simulink model "Ej11"  (R2025b)
settings: Solver=VariableStepAuto  StartTime=0.0  StopTime=inf  RelTol=1e-3
libraries: commdigbbndam3 x4, commrandsrc3 x1
settings Model: Creator=Henry  LastModifiedBy=Henry

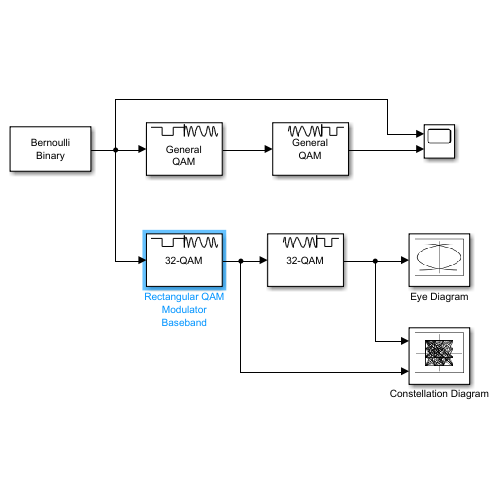
[thumbnail: Simulink's stored preview of the top-level diagram]
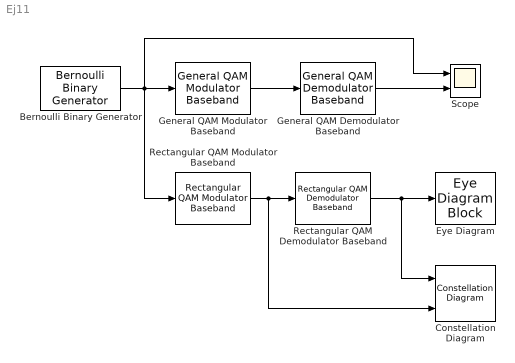
== system Ej11 ==
  Bernoulli Binary Generator : commrandsrc3/Bernoulli Binary Generator  ProbabilityOfZero=0.5  SeedSource=Auto  Seed=0  SampleTime=1  SamplesPerFrame=2  OutputDataType=double  SimulateUsing=Interpreted execution
  Constellation Diagram : ConstellationDiagram  NumInputPorts=2  WindowPosition=[36.000000,127.000000,600.000000,600.000000,]  ScopeFrameLocation=window  SymbolsToDisplay=8  ReferenceConstellation="{[-1.0801+1.0801i         -1.0801+0.77152i         -1.0801+0.46291i          -1.0801+0.1543i          -1.0801-0.1543i         -1.0801-0.46291i         -1.0801-0.77152i          -1.0801-1.0801i         -0.77152+1.0801i        -0.77152+0.77152i        -0.77152+0.46291i         -0.77152+0.1543i         -0.77152-0.1543i        -0.77152-0.46291i        -0.77152-0.77152i         -0.77152-1.0801i         -0.46291+1.0801i        -0.46291+0.77152i        -0.46291+0.46291i         -0.46291+0.1543i         -0.46291-0.1543i        -0.46291-0.46291i        -0.46291-0.77152i         -0.46291-1.0801i          -0.1543+1.0801i         -0.1543+0.77152i         -0.1543+0.46291i          -0.1543+0.1543i          -0.1543-0.1543i         -0.1543-0.46291i         -0.1543-0.77152i          -0.1543-1.0801i           0.1543+1.0801i          0.1543+0.77152i          0.1543+0.46291i           0.1543+0.1543i           0.1543-0.1543i          0.1543-0.46291i          0.1543-0.77152i           0.1543-1.0801i          0.46291+1.0801i         0.46291+0.77152i         0.46291+0.46291i          0.46291+0.1543i          0.46291-0.1543i         0.46291-0.46291i         0.46291-0.77152i          0.46291-1.0801i          0.77152+1.0801i         0.77152+0.77152i         0.77152+0.46291i          0.77152+0.1543i          0.77152-0.1543i         0.77152-0.46291i         0.77152-0.77152i          0.77152-1.0801i           1.0801+1.0801i          1.0801+0.77152i          1.0801+0.46291i           1.0801+0.1543i           1.0801-0.1543i          1.0801-0.46291i          1.0801-0.77152i           1.0801-1.0801i][-1.0801+1.0801i         -1.0801+0.77152i         -1.0801+0.46291i          -1.0801+0.1543i          -1.0801-0.1543i         -1.0801-0.46291i         -1.0801-0.77152i          -1.0801-1.0801i         -0.77152+1.0801i        -0.77152+0.77152i        -0.77152+0.46291i         -0.77152+0.1543i         -0.77152-0.1543i        -0.77152-0.46291i        -0.77152-0.77152i         -0.77152-1.0801i         -0.46291+1.0801i        -0.46291+0.77152i        -0.46291+0.46291i         -0.46291+0.1543i         -0.46291-0.1543i        -0.46291-0.46291i        -0.46291-0.77152i         -0.46291-1.0801i          -0.1543+1.0801i         -0.1543+0.77152i         -0.1543+0.46291i          -0.1543+0.1543i          -0.1543-0.1543i         -0.1543-0.46291i         -0.1543-0.77152i          -0.1543-1.0801i           0.1543+1.0801i          0.1543+0.77152i          0.1543+0.46291i           0.1543+0.1543i           0.1543-0.1543i          0.1543-0.46291i          0.1543-0.77152i           0.1543-1.0801i          0.46291+1.0801i         0.46291+0.77152i         0.46291+0.46291i          0.46291+0.1543i          0.46291-0.1543i         0.46291-0.46291i         0.46291-0.77152i          0.46291-1.0801i          0.77152+1.0801i         0.77152+0.77152i         0.77152+0.46291i          0.77152+0.1543i          0.77152-0.1543i         0.77152-0.46291i         0.77152-0.77152i          0.77152-1.0801i           1.0801+1.0801i          1.0801+0.77152i          1.0801+0.46291i           1.0801+0.1543i           1.0801-0.1543i          1.0801-0.46291i          1.0801-0.77152i           1.0801-1.0801i]}"  ShowLegend=on  ShowTrajectory=on
  Eye Diagram : EyeDiagramBlock  WindowPosition=[666.000000,186.000000,800.000000,500.000000,]  ScopeFrameLocation=window  YLimits=[-1.1,1.125]
  General QAM Demodulator Baseband : commdigbbndam3/General QAM Demodulator Baseband  SigCon=[exp(2*pi*1i*[0:7]/8)]  OutType=Integer  DecType=Hard decision  VarSource=Dialog  Variance=1  outDtypeBit=Inherit via internal rule  outDtype=Inherit via internal rule  roundingMode=Floor  overflowMode=Wrap  OvFlMode=off  OvFlModeLastStrValue=off  sigConstWordLen=16  sigConstDataTypeStr=Inherit: Same word length as input  sigConstLastDataTypeStr=Inherit: Same word length as input  accum1WordLen=32  accum1FracLen=30  prodInWordLen=32  prodInFracLen=30  prodInDataTypeStr=Inherit: Same as accumulator 1  prodInLastDataTypeStr=Inherit: Same as accumulator 1  prodOutWordLen=32  prodOutFracLen=30  accum2WordLen=32  accum2FracLen=30  accum3WordLen=32  accum3FracLen=30  nsiWordLen=32  nsiFracLen=30  nsiDataTypeStr=Inherit: Same as accumulator 3  nsiLastDataTypeStr=Inherit: Same as accumulator 3  invn0WordLen=16  invn0FracLen=8  invn0DataTypeStr=Inherit: Same word length as input  invn0LastDataTypeStr=Inherit: Same word length as input  outputWordLen=32  outputFracLen=30
  General QAM Modulator Baseband : commdigbbndam3/General QAM Modulator Baseband  SigCon=[exp(2*pi*1i*[0:7]/8)]  outDtype=double  outWordLen=16  outUDDataType=sfix(16)  outFracLenMode=Best precision  outFracLen=15  outDataTypeStr=double  outLastDataTypeStr=double
  Rectangular QAM Demodulator Baseband : commdigbbndam3/Rectangular QAM Demodulator Baseband  M=32  OutType=Integer  DecType=Hard decision  VarSource=Dialog  Variance=1  Dec=Gray  Mapping=[0:15]  PowType=Min. distance between symbols  MinDist=2  AvgPow=1  PeakPow=1  Ph=0  outDtype1=Inherit via internal rule  outDtype2=Inherit via internal rule  derotateFactorWordLen=16  derotateFactorDataTypeStr=Inherit: Same word length as input  derotateFactorLastDataTypeStr=Inherit: Same word length as input  denormFactorWordLen=16  denormFactorDataTypeStr=Inherit: Same word length as input  denormFactorLastDataTypeStr=Inherit: Same word length as input  prodOutWordLen=32  prodOutOverflowMode=Wrap  prodOutRoundingMode=Floor  prodOutOvFlMode=off  prodOutOvFlModeLastStrValue=off  sumWordLen=32
  Rectangular QAM Modulator Baseband : commdigbbndam3/Rectangular QAM Modulator Baseband  M=32  InType=Integer  Enc=Gray  Mapping=[0:15]  PowType=Min. distance between symbols  MinDist=2  AvgPow=1  PeakPow=1  Ph=0  outDtype=double  outWordLen=16  outUDDataType=sfix(16)  outFracLenMode=Best precision  outFracLen=15  outDataTypeStr=double  outLastDataTypeStr=double
  Scope : Scope  NumInputPorts=2
      settings: ActiveDisplayYMinimum=-1  ActiveDisplayYMaximum=1
  wires:
  Bernoulli Binary Generator/1 -> Scope/1, Rectangular QAM Modulator Baseband/1, General QAM Modulator Baseband/1
  General QAM Modulator Baseband/1 -> General QAM Demodulator Baseband/1
  Rectangular QAM Modulator Baseband/1 -> Constellation Diagram/2, Rectangular QAM Demodulator Baseband/1
  General QAM Demodulator Baseband/1 -> Scope/2
  Rectangular QAM Demodulator Baseband/1 -> Constellation Diagram/1, Eye Diagram/1
